simulink model "pll2ins_simulink"  (R2021a)
settings: Solver=ode4  StartTime=0.0  StopTime=1.0  FixedStep=0.001  RelTol=1e-3
settings Model: Creator=longt  LastModifiedBy=longt
settings DataIOCC: SaveOutput=off  SignalLogging=off  DSMLogging=off  SaveTime=off  ReturnWorkspaceOutputs=off

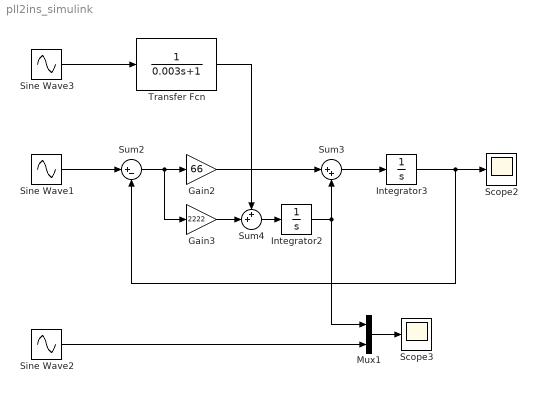
== system pll2ins_simulink ==
  Gain2 : Gain  Gain=66
  Gain3 : Gain  Gain=2222
  Integrator2 : Integrator
  Integrator3 : Integrator
  Mux1 : Mux  Inputs=2
  Scope2 : Scope
  Scope3 : Scope
  Sine Wave1 : Sin  Frequency=10*2*pi  SampleTime=0
  Sine Wave2 : Sin  Amplitude=10*2*pi  Frequency=10*2*pi  Phase=pi/2  SampleTime=0
  Sine Wave3 : Sin  Amplitude=(10*2*pi)^2  Frequency=10*2*pi  Phase=pi  SampleTime=0
  Sum2 : Sum  Inputs=|+-
  Sum3 : Sum  Inputs=|++
  Sum4 : Sum  Inputs=++|
  Transfer Fcn : TransferFcn  Denominator=[0.003 1]
  wires:
  Mux1/1 -> Scope3/1
  Integrator3/1 -> Scope2/1, Sum2/2
  Sum3/1 -> Integrator3/1
  Integrator2/1 -> Sum3/2, Mux1/1
  Gain2/1 -> Sum3/1
  Sum2/1 -> Gain2/1, Gain3/1
  Sine Wave1/1 -> Sum2/1
  Gain3/1 -> Sum4/2
  Sum4/1 -> Integrator2/1
  Transfer Fcn/1 -> Sum4/1
  Sine Wave2/1 -> Mux1/2
  Sine Wave3/1 -> Transfer Fcn/1
